simulink model "Drone_NAV_SLAM"  (R2024a)
settings: Solver=FixedStepAuto  StartTime=0.0  StopTime=inf  RelTol=1e-3
libraries: robotcorelib x3, uavutilslib x2
settings Model: Creator=quentinlandon  LastModifiedBy=quentinlandon
settings SolverCC: AllowMultiTaskInputOutput=on  ConcurrentTasks=on

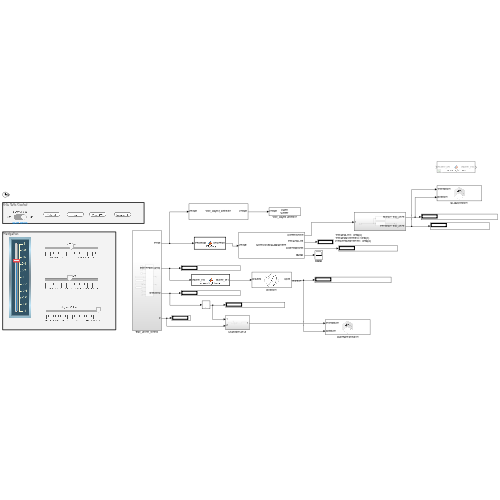
[thumbnail: Simulink's stored preview of the top-level diagram]
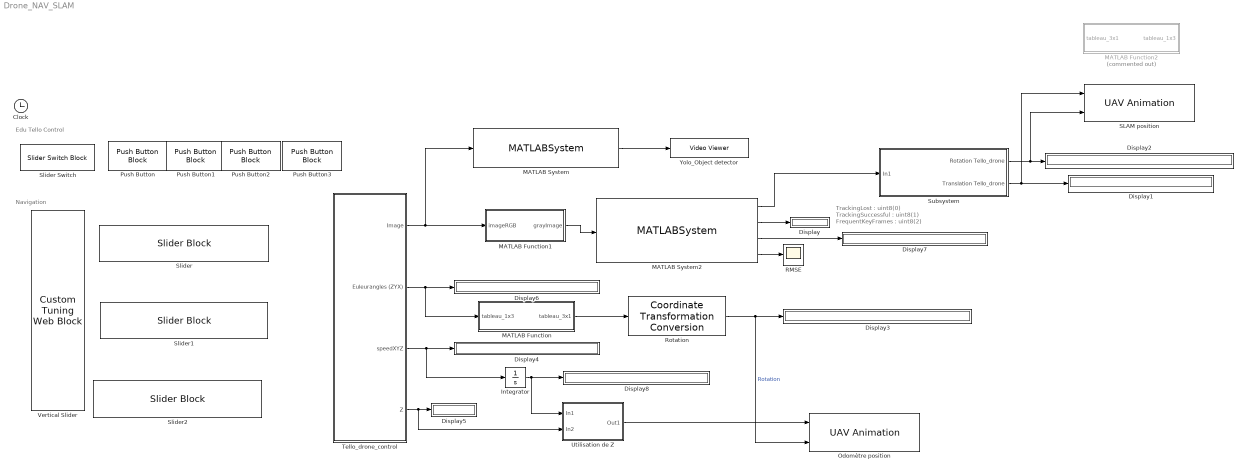
== system Drone_NAV_SLAM ==
  note: TrackingLost : uint8(0)
      | TrackingSuccessful : uint8(1)
      | FrequentKeyFrames : uint8(2)
  note: Navigation
  note: Edu Tello Control
  Clock : Clock
  Display{,1..8} (9 alike) : Display
  Integrator : Integrator
  MATLAB Function : MATLAB Function  TreatAsAtomicUnit=on
  MATLAB Function1 : MATLAB Function  TreatAsAtomicUnit=on
  MATLAB Function2 : MATLAB Function  Commented=on  TreatAsAtomicUnit=on
  MATLAB System : MATLABSystem  System=Yolo_Object_Detector  SimulateUsing=Interpreted execution
      mask Type: Yolo_Object_Detector
      mask Display:
      | disp('Yolo_Object_Detector');
      | port_label('input',1,'Image');
      | port_label('output',1,'Image');
  MATLAB System2 : MATLABSystem  System=MonoVisualSLAMSystem  FocalLength=[ 657, 650 ]  PrincipalPoint=[ 501, 427 ]  ImageSize=[ 720, 960 ]  SimulateUsing=Interpreted execution
      mask Type: MonoVisualSLAMSystem
      mask Display:
      | disp('MonoVisualSLAMSystem');
      | port_label('input',1,'Image');
      | port_label('output',1,'Camera Pose');
      | port_label('output',2,'Tracking Lost');
      | port_label('output',3,'XYZmappoints');
      | port_label('output',4,'RMSE');
  Odomètre position : uavutilslib/UAV Animation  UAVType=Multirotor  UAVSize=1  InertialZDirection=Up  SampleTime=-1
  Push Button : PushButtonBlock  ButtonText=Takeoff  OffValue=0.000000
  Push Button1 : PushButtonBlock  ButtonText=Land  OffValue=0.000000
  Push Button2 : PushButtonBlock  ButtonText=MoveXYZ  OffValue=0.000000
  Push Button3 : PushButtonBlock  ButtonText=Moverotate  OffValue=0.000000
  RMSE : Scope
  Rotation : robotcorelib/Coordinate Transformation Conversion  InputRepresentation=Euler Angles  InputEulerSequence=ZYX  ShowTrVecInputPort=on  OutputRepresentation=Quaternion  OutputEulerSequence=ZYX  ShowTrVecOutputPort=off  SimulateUsing=Code generation
      settings: LibrarySourceBlock=uavutilslib/Coordinate Transformation Conversion
  SLAM position : uavutilslib/UAV Animation  UAVType=Multirotor  UAVSize=1  InertialZDirection=Down  SampleTime=-1
  Slider : SliderBlock  ScaleMin=-1  ScaleMax=1
  Slider Switch : SliderSwitchBlock
      settings: Values={{'Off', 'On'}, [0 1]}
  Slider1 : SliderBlock  ScaleMin=-1  ScaleMax=1
  Slider2 : SliderBlock  ScaleMin=-180  ScaleMax=180
  Subsystem : Subsystem
  Tello_drone_control : Subsystem
  Utilisation de Z : Subsystem
  Vertical Slider : CustomTuningWebBlock  LabelPosition=Hide  ShowInitialText=on  Configuration="{\"components\":[{\"name\":\"LinearScaleComponent\",\"settings\":{\"bounds\":{\"max\":1,\"min\":-1,\"tickInterval\":\"auto\"},\"internalTickHeightScaleFactor\":0.5,\"labelColor\":[255,255,200],\"labelFont\":{\"font\":\"Arial\",\"fontSize\":12},\"labelOffset\":0.05,\"labelTransparency\":1,\"needleImage\":{\"size\":[596,842],\"src\":\"data:image\\/svg+xml;base64,PD94bWwgdmVyc2lvbj0iMS4wIiBlbmNvZGluZz0idXRmLTgiPz4NCjwhLS0gR2VuZXJhdG9yOiBBZG9iZSBJbGx1c3RyYXRvciAyNS4wLjAsIFNWRyBFeHBvcnQgUGx1Zy1JbiAuIFNWRyBWZXJzaW9uOiA2LjAwIEJ1aWxkIDApICAtLT4NCjxzdmcgdmVyc2lvbj0iMS4xIg0KCSBpZD0ic3ZnOCIgeG1sbnM6Y2M9Imh0dHA6Ly9jcmVhdGl2ZWNvbW1vbnMub3JnL25zIyIgeG1sbnM6ZGM9Imh0dHA6Ly9wdXJsLm9yZy9kYy9lbGVtZW50cy8xLjEvIiB4bWxuczppbmtzY2FwZT0iaHR0cDovL3d3dy5pbmtzY2FwZS5vcmcvbmFtZXNw ...(+2420 chars)\",\"srcOrientation\":\"horizontal\"},\"needleOffset\":[0.0642123287671233,-0.8044596912521441],\"needleSize\":{\"height\":0.07668067226890757,\"width\":0.4337797619047619},\"position\":[0.03623949579831933,0.2829861111111111,0.6088789682539683,0.9196428571428571],\"referencePoint\":\"auto\",\"scaleColors\":[],\"scaleColorsSize\":0.2,\"scaleDirection\":\"BT\",\"showLabels\":1,\"showMinorTicks\":0,\"showSpanLine\":1,\"showTicks\":1,\"tickColor\":[252,252,197],\"tickTransparency\":1,\"valueBarColor\":[0,114,189],\"valueBarOffset\":-0.27,\"valueBarSize\":0.1,\"valueBarTransparency\":1}},{\"name\":\"BackgroundImageComponent\",\"settings\":{\"image\":{\"size\":[380,101],\"src\":\"data:image\\/svg+xml;base64,PHN2ZyB4bWxucz0iaHR0cDovL3d3dy53My5vcmcvMjAwMC9zdmciIHhtbG5zOnhsaW5rPSJodHRwOi8vd3d3LnczLm9yZy8xOTk5L3hsaW5rIiB2aWV3Qm94PSIwIDAgMzgwIDEwMSI+PGRlZnM+PHN0eWxlPi5jbHMtMXtmaWxsOiMwMDJiNDI7fS5jbHMtMntmaWxsOiM0MjcwODI7fS5jbHMtM3tmaWxsOnVybCgjcmFkaWFsLWdyYWRpZW50KTt9LmNscy00e2ZpbGw6I2M4YzhjODtzdHJva2U6IzAwMDt9PC9zdHlsZT48cmFkaWFsR3JhZGllbnQgaWQ9InJhZGlhbC1ncmFkaWVudCIgY3g9IjE5MCIgY3k9IjUwLjUiIHI9IjI2OS4yMSIgZ3JhZGllbnRVbml0cz0idXNlclNwYWNlT25Vc2UiPjxzdG9wIG9mZnNldD0iMC4wMSIgc3RvcC1jb2xvcj0iIzNlNGY1OCIvPjxzdG9wIG9mZnNldD0iMC4wNiIgc3RvcC1jb2xvcj0iIzQ0NTc2MSIvPjxzdG9wIG9mZnNldD0iMC4xNSIgc3RvcC1jb2xvcj0iIzU1NmE3NiIvPjxzdG9wIG9mZnNldD0iMC4yNSIgc3RvcC1jb2xvcj0iIzZkODg5NSIvPjxzdG9wIG9mZnNldD0iMC4zOCIgc3RvcC1jb2xvcj0iIzhmYjJjMyIvPjxzdG9wIG9mZnNldD0iMC41MiIgc3RvcC1jb2xvcj0iI2I2ZTRmYSIvPjxzdG9wIG9mZnNldD0iMSIgc3RvcC1jb2xvcj0iIzE1NDY1NyIvPjwvcmFkaWFsR3JhZGllbnQ+PC9kZWZzPjxnIGlkPSJmcmFtZSI+PGcgaWQ9IkxheWVyXzIiIGRhdGEtbmFtZT0iTGF5ZXIgMiI+PGcgaWQ9IkxheWVyXzEtMiIgZGF0YS1uYW1lPSJMYXllciAxLTIiPjxyZWN0IGlkPSJyZWN0MTAzNiIgY2xhc3M9ImNscy0xIiB4PSIxMSIgeT0iMTEiIHdpZHRoPSIzNTgiIGhlaWdodD0iNzkiLz48cGF0aCBpZD0icGF0aDEwMzgiIGNsYXNzPSJjbHMtMiIgZD0iTTgsOFY5M0gzNzJWOFpNMzY5LDkwSDExVjExSDM2OVoiLz48cGF0aCBpZD0icGF0aDEwNDAiIGNsYXNzPSJjbHMtMyIgZD0iTTAsMFYxMDFIMzgwVjBaTTM3Miw5M0g4VjhIMzcyWiIvPjwvZz48L2c+PC9nPjxnIGlkPSJ0cmFjayI+PHBhdGggaWQ9InJlY3QxNjExIiBjbGFzcz0iY2xzLTQiIGQ9Ik0zMy4zNywyNi41OUgzNDYuNjNjNCwwLDcuMjUsMi42LDcuMjUsNS44MWgwYzAsMy4yMS0zLjI1LDUuODItNy4yNSw1LjgySDMzLjM3Yy00LDAtNy4yNS0yLjYxLTcuMjUtNS44MmgwQzI2LjEyLDI5LjE5LDI5LjM3LDI2LjU5LDMzLjM3LDI2LjU5WiIvPjwvZz48L3N2Zz4=\",\"srcOrientation\":\"horizontal\"},\"position\":[0,0,1,1],\"scaleMode\":\"0\"}},{\"name\":\"ForegroundImageComponent\",\"settings\":{\"image\":{\"size\":[0,0],\"src\":\"default\",\"srcOrientation\":[]},\"isForeground\":1,\"position\":[0,0,1,1],\"scaleMode\":\"0\"}}],\"settings\":{\"BindingType\":\"param\",\"aspectRatio\":3.7777777777777777,\"backgroundColor\":[0,0,0,\"1\"],\"backgroundOffset\":0,\"backgroundOpacity\":1,\"fixedAspectRatio\":\"on\",\"foregroundColor\":[252,252,196],\"orientation\":\"vertical\",\"showBackgroundColor\":false,\"value\":0,\"version\":\"R2023a\"},\"type\":\"LinearGauge\"}"
  Yolo_Object detector : VideoViewer  FigPos=[2672 616 627 444]
  wires:
  MATLAB Function1/1(grayImage) -> MATLAB System2/1
  MATLAB System/1 -> Yolo_Object detector/1
  Tello_drone_control/1(Image) -> MATLAB Function1/1(imageRGB), MATLAB System/1
  MATLAB System2/2 -> Display/1
  MATLAB System2/1 -> Subsystem/1(In1)
  Subsystem/1(Rotation Tello_drone) -> SLAM position/2, Display2/1
  Subsystem/2(Translation Tello_drone) -> SLAM position/1, Display1/1
  Tello_drone_control/2(Euleurangles (ZYX)) -> Display6/1, MATLAB Function/1(tableau_1x3)
  Rotation/1 -> Display3/1, Odomètre position/2  "Rotation"
  Tello_drone_control/3(speedXYZ) -> Integrator/1, Display4/1
  Tello_drone_control/4(Z) -> Utilisation de Z/2(In2), Display5/1
  MATLAB Function/1(tableau_3x1) -> Rotation/1
  MATLAB System2/3 -> Display7/1
  Integrator/1 -> Utilisation de Z/1(In1), Display8/1
  Utilisation de Z/1(Out1) -> Odomètre position/1
  MATLAB System2/4 -> RMSE/1

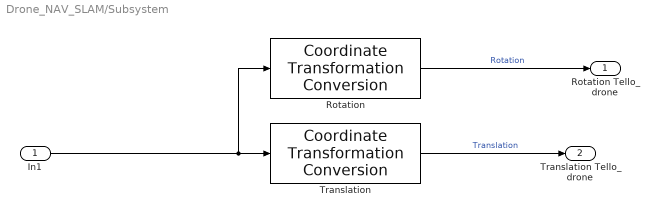
== system Drone_NAV_SLAM/Subsystem ==
  In1 : Inport
  Rotation : robotcorelib/Coordinate Transformation Conversion  InputRepresentation=Homogeneous Transformation  InputEulerSequence=ZYX  ShowTrVecInputPort=on  OutputRepresentation=Quaternion  OutputEulerSequence=ZYX  ShowTrVecOutputPort=off  SimulateUsing=Code generation
      settings: LibrarySourceBlock=uavutilslib/Coordinate Transformation Conversion
  Translation : robotcorelib/Coordinate Transformation Conversion  InputRepresentation=Homogeneous Transformation  InputEulerSequence=ZYX  ShowTrVecInputPort=on  OutputRepresentation=Translation Vector  OutputEulerSequence=ZYX  ShowTrVecOutputPort=on  SimulateUsing=Code generation
      settings: LibrarySourceBlock=uavutilslib/Coordinate Transformation Conversion
  Rotation Tello_drone : Outport
  Translation Tello_drone : Outport  Port=2
  wires:
  Translation/1 -> Translation Tello_drone/1  "Translation"
  Rotation/1 -> Rotation Tello_drone/1  "Rotation"
  In1/1 -> Rotation/1, Translation/1

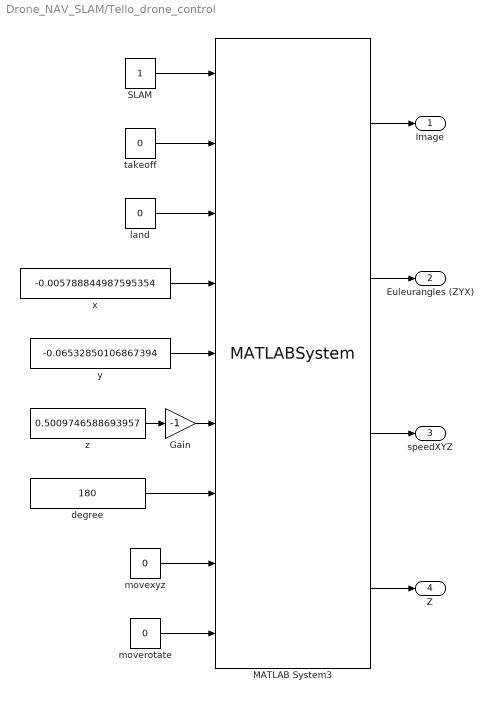
== system Drone_NAV_SLAM/Tello_drone_control ==
  Gain : Gain  Gain=-1
  MATLAB System3 : MATLABSystem  System=Tello_drone_control  droneIP=127.0.0.1  SimulateUsing=Interpreted execution
      mask Type: Tello_drone_control
      mask Display:
      | disp('Tello_drone_control');
      | port_label('input',1,'Slam');
      | port_label('input',2,'tkoff');
      | port_label('input',3,'landing');
      | port_label('input',4,'xMove');
      | port_label('input',5,'yMove');
      | port_label('input',6,'zMove');
      | port_label('input',7,'degree');
      | port_label('input',8,'movexyz');
      | port_label('input',9,'moverotate');
      | port_label('output',1,'image');
      | port_label('output',2,'Eulerangles');
      | port_label('output',3,'speedXYZ');
      | port_label('output',4,'height');
  SLAM : Constant
  degree : Constant  Value=180
  land : Constant  Value=0
  moverotate : Constant  Value=0
  movexyz : Constant  Value=0
  takeoff : Constant  Value=0
  x : Constant  Value=-0.005788844987595354
  y : Constant  Value=-0.06532850106867394
  z : Constant  Value=0.5009746588693957
  Image : Outport
  Euleurangles (ZYX) : Outport  Port=2
  speedXYZ : Outport  Port=3
  Z : Outport  Port=4
  wires:
  moverotate/1 -> MATLAB System3/9
  land/1 -> MATLAB System3/3
  y/1 -> MATLAB System3/5
  x/1 -> MATLAB System3/4
  Gain/1 -> MATLAB System3/6
  z/1 -> Gain/1
  degree/1 -> MATLAB System3/7
  SLAM/1 -> MATLAB System3/1
  movexyz/1 -> MATLAB System3/8
  MATLAB System3/1 -> Image/1
  takeoff/1 -> MATLAB System3/2
  MATLAB System3/2 -> Euleurangles (ZYX)/1
  MATLAB System3/3 -> speedXYZ/1
  MATLAB System3/4 -> Z/1

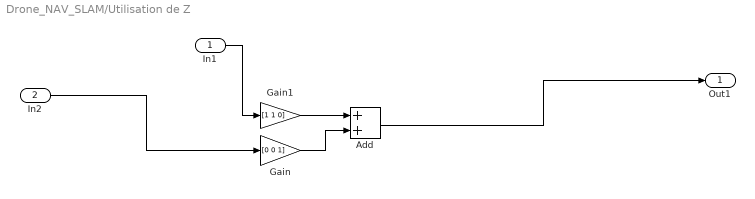
== system Drone_NAV_SLAM/Utilisation de Z ==
  In1 : Inport
  In2 : Inport  Port=2
  Add : Sum
  Gain : Gain  Gain=[0 0 1]
  Gain1 : Gain  Gain=[1 1 0]
  Out1 : Outport
  wires:
  Add/1 -> Out1/1
  In1/1 -> Gain1/1
  In2/1 -> Gain/1
  Gain1/1 -> Add/1
  Gain/1 -> Add/2

== matlab function Drone_NAV_SLAM/MATLAB Function ==
  data: tableau_1x3 input; tableau_3x1 output
function tableau_3x1  = convertir_tableau(tableau_1x3)
    tableau_3x1 = tableau_1x3';
end

== matlab function Drone_NAV_SLAM/MATLAB Function2 ==
  data: tableau_3x1 input; tableau_1x3 output
function tableau_1x3  = convertir_tableau(tableau_3x1)
    tableau_1x3 = tableau_3x1';
    
end

== matlab function Drone_NAV_SLAM/MATLAB Function1 ==
  data: imageRGB input; grayImage output
function grayImage = rgbToGray(imageRGB)
    grayImage = rgb2gray(imageRGB);
end
